simulink model "E1_1"  (R2021a)
settings: Solver=VariableStepAuto  StartTime=0.0  StopTime=100  RelTol=1e-3
settings Model: Creator=erlen  LastModifiedBy=erlen

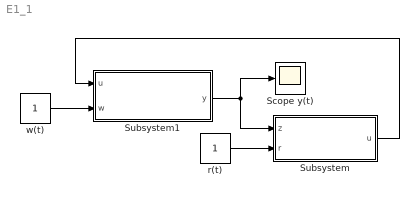
== system E1_1 ==
  Scope y(t) : Scope
  Subsystem : Subsystem
  Subsystem1 : Subsystem
  r(t) : Constant
  w(t) : Constant
  wires:
  Subsystem1/1(y) -> Scope y(t)/1, Subsystem/1(z)
  Subsystem/1(u) -> Subsystem1/1(u)
  w(t)/1 -> Subsystem1/2(w)
  r(t)/1 -> Subsystem/2(r)

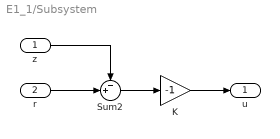
== system E1_1/Subsystem ==
  z : Inport
  r : Inport  Port=2
  K : Gain  Gain=-1
  Sum2 : Sum  Inputs=-+|
  u : Outport
  wires:
  Sum2/1 -> K/1
  r/1 -> Sum2/2
  K/1 -> u/1
  z/1 -> Sum2/1

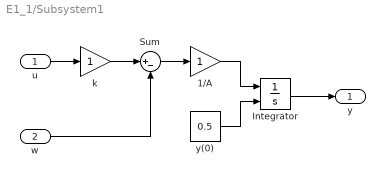
== system E1_1/Subsystem1 ==
  u : Inport
  w : Inport  Port=2
  1/A : Gain
  Integrator : Integrator  InitialConditionSource=external
  Sum : Sum  Inputs=|+-
  k : Gain
  y(0) : Constant  Value=0.5
  y : Outport
  wires:
  k/1 -> Sum/1
  w/1 -> Sum/2
  u/1 -> k/1
  y(0)/1 -> Integrator/2
  Sum/1 -> 1/A/1
  1/A/1 -> Integrator/1
  Integrator/1 -> y/1
